simulink model "may20EOD"  (R2019b)
settings: Solver=ode4  StartTime=0.0  StopTime=inf  FixedStep=BKIN_STEP_TIME  RelTol=1e-3  EnableMultiTasking=on
StartFcn:
  |  warndlg('Dexterit-E models cannot run under simulation. Please compile your model and run it from within Dexterit-E.');set_param(bdroot,'SimulationCommand','stop')
model workspace (MAT data in the model file):
  BARRIER_ROW = 5
  BKIN_KINEMATIC_FRAME_SIZE = 400
  BKIN_STEP_TIME = 0.00025
  CIRCLE_STROKE = 10
  CIRCLE_STROKE_W = 11
  CURSOR_ROW = 2
  E_BARRIER_HIT = 6
  E_COLLISION_HIT = 7
  E_ENTER_PRESHOT_AREA = 2
  E_ENTER_START_AREA = 12
  E_EXIT = 13
  E_EXIT_PRESHOT_AREA = 10
  E_GOAL_HIT = 8
  E_GOAL_REACHED = 5
  E_NO_EVENT = 0
  E_PRESHOT_ROW = 4
  E_TARGET_OUT_OF_BOUNDS = 9
  E_TRIAL_BEGIN = 1
  E_TRIAL_ENDED = 3
  FIRST_FILL = 8
  FORCE_MULTIPLIER = 1
  F_BUMP = 1
  GOAL_ROW = 8
  GOAL_TIME = 12
  HEIGHT = 6
  INVISIBLE_FILL = 15
  LOAD_ROW = 4
  MASS_CIRCLE = 2
  MASS_RECT = 3
  PERT_DUR = 5
  PERT_RAMP = 4
  PRESHOT_ROW = 7
  PUCK_ROW = 3
  RADIUS_LOG = 4
  RADIUS_VIS = 5
  RECT_STROKE = 13
  RECT_STROKE_W = 14
  ROTATION = 7
  SECONDS = 1
  SECOND_FILL = 9
  SHOT_READY_TIME = 10
  SHOT_SET_TIME = 11
  START_HOLD_TIME = 9
  START_ROW = 6
  THIRD_FILL = 12
  TRIAL_FAILURE = 11
  WIDTH = 3
  col_x = 1
  col_y = 2
undefined symbols (not defined in the file): slselsubs
libraries: Video x7, General x3, KINARM_loads x2, KINARM_EP_loads x1, KINARM_general x1, simulink x1, slrtlib x1
(part 1 of 3)
settings Model: ModifiedComment=chris -- Wed Feb 16 09:18:30 2005 -- Version 1.1384  ModifiedHistory=Feb 16/05 - Add error repeat, add offset ramp  ExtModeArmWhenConnect=off  ExtModeLogAll=off  OrderedModelArguments=off  Creator=Chris Grebeldinger  LastModifiedBy=User
settings SolverCC: AutoInsertRateTranBlk=on
settings DataIOCC: SaveFormat=Array  SignalLoggingSaveFormat=ModelDataLogs  SaveOutput=off  SaveTime=off  ReturnWorkspaceOutputs=off  SignalLoggingName=sigsOut
settings OptimizationCC: BlockReduction=off  BooleanDataType=off  OptimizeBlockIOStorage=off  BufferReuse=off  GlobalBufferReuse=off  ExpressionFolding=off  ExpressionDepthLimit=2147483647  LocalBlockOutputs=off  InitFltsAndDblsToZero=on  LifeSpan=inf  OptimizeDataStoreBuffers=off  BusAssignmentInplaceUpdate=off
settings DebuggingCC: SaveWithParameterizedLinksMsg=none  UnderspecifiedInitializationDetection=Classic  MergeDetectMultiDrivingBlocksExec=none  SignalResolutionControl=TryResolveAllWithWarning  MultiTaskDSMMsg=warning  FcnCallInpInsideContextMsg=warning  BusObjectLabelMismatch=none  StateNameClashWarn=warning  StrictBusMsg=ErrorOnBusTreatedAsVector  SFUnexpectedBacktrackingDiag=warning  SFNoUnconditionalDefaultTransitionDiag=warning  SFExecutionAtInitializationDiag=none  ArithmeticOperatorsInVariantConditions=warning
settings HardwareCC: ProdBitPerPointer=32  ProdBitPerSizeT=32  ProdBitPerPtrDiffT=32  ProdLargestAtomicFloat=None  ProdWordSize=32  ProdLongLongMode=on  ProdHWDeviceType=Generic->32-bit x86 compatible  TargetHWDeviceType=32-bit Generic
settings ModelReferenceCC: PropagateSignalLabelsOutOfModel=off
settings SFSimCC: SimUseLocalCustomCode=off  SimParseCustomCode=off  CustomCodeUndefinedFunction=UseInterfaceOnly
settings RTWCC: Description=Simulink Real-Time  SystemTargetFile=slrt.tlc  TemplateMakefile=slrt_default_tmf  RTWUseLocalCustomCode=off  CodeExecutionProfiling=on  RTWCompilerOptimization=on
settings CodeAppCC: MaxIdLength=63  StateflowObjectComments=on
settings SimulinkRealTimeCC: TargetFcnLib=ansi_tfl_tmw.mat  GeneratePreprocessorConditionals=Disable all  PreserveStateflowLocalDataDimensions=off
settings ConfigComp: CovMetricSettings=dw  CovHtmlReporting=on  CovSaveCumulativeToWorkspaceVar=on  CovSaveSingleToWorkspaceVar=on  CovExternalEMLEnable=off

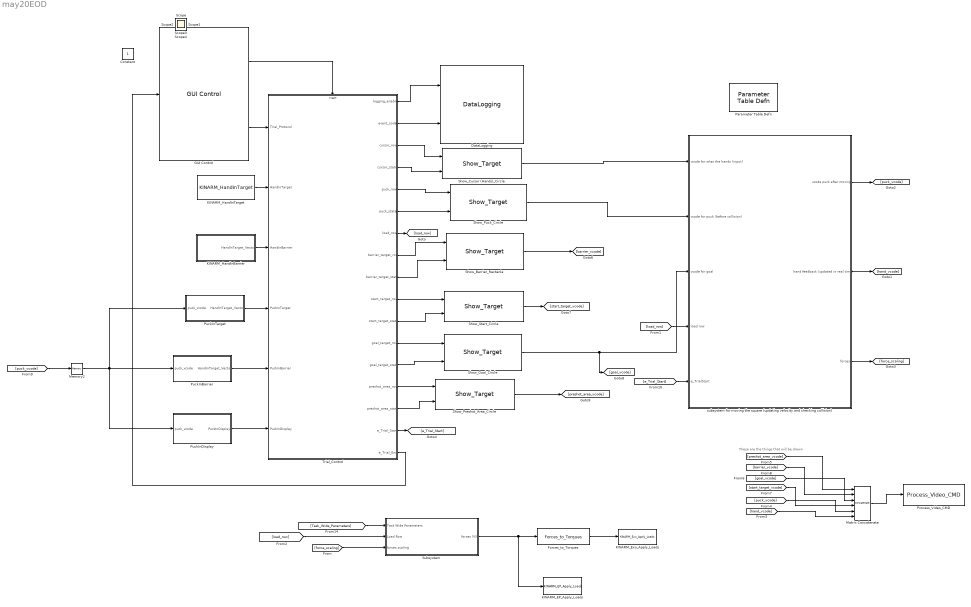
== system may20EOD ==
  note: These are the things that will be drawn
  DataLogging : General/DataLogging  log_event_codes=on  log_analog_inputs=off  show_time_remaining=off  ecat_include=on
  Forces_to_Torques : KINARM_loads/Forces_to_Torques
  GUI Control : General/GUI Control  task_version=1.0  show_repeat_trial_flag=off  use_custom_tp=off  target_type_str=Circle  Target_Type=1  XYcols=[1 2]  Vcols=3  Lcols=4  indices_padding=[0 0 0 0;0 0 0 0]  target_table_rows=64  load_table_rows=20  tp_table_rows=100
  KINARM_EP_Apply_Loads : KINARM_EP_loads/KINARM_EP_Apply_Loads  up_duration=1500  down_duration=1500  max_force=20
  KINARM_Exo_Apply_Loads : KINARM_loads/KINARM_Exo_Apply_Loads  up_duration=1500  down_duration=1500  max_torque=5  limit_motors=off
  KINARM_HandInBarrier : Subsystem  AncestorBlock=KINARM_general/KINARM_HandInTarget  mask(KINARM_HandInTarget){use_dominant_hand=on, target_type=Rectangle, num_states=1, attribcol1=[WIDTH HEIGHT ROTATION], attribcol2=[0 0 0], attribcol3=[0 0 0], attribcol4=[0 0 0], attribcol5=[0 0 0]}
      mask prompts: use_dominant_hand "Use "arm to be assessed"?"; target_type "Type of Target"; num_states "Number of Target States"; attribcol1 "State 1 Target Table Column(s)"; attribcol2 "State 2 Target Table Column(s)"; attribcol3 "State 3 Target Table Column(s)"; attribcol4 "State 4 Target Table Column(s)"; attribcol5 "State 5 Target Table Column(s)"
      mask help: This block returns a vector or array corresponding to the Target_Table rows indicating whether the specified hand is in (=1) or out (=0) of each of the targets.
      mask init:
      | block_path = gcb;  % store block path, as gcb may change with block operations
      | 
      | %%% Get the model's workspace, because it is required to evaluate constants from the Parameter Table Def'n block
      | modelName=bdroot(block_path);
      | modelWorkspace = get_param(modelName, 'ModelWorkspace');
      | 
      | %%% Handle background colours if link status changes.  
      | checkBackgroundColour(block_path, 'KINARM_general');
      | 
      | %%% create the names of the input and output ports to display on the mask
      | % Select only the desired states for output. The output port is also renamed to reflect 
      | % whether the output is a vector (in the case of a single state) or an array (of vectors, 
      | % one for each of multiple states).
      | 
      | numStates = str2double( get_param(block_path, 'num_states') );
      | 
      | if numStates == 1
      | 	set_param([block_path '/Selected States'], 'Value', '[1]');
      | 	outputname = 'HandInTarget_Vector';
      | elseif numStates == 2
      | 	set_param([block_path '/Selected States'], 'Value', '[1,2]');
      | 	outputname = 'HandInTarget_Array';
      | elseif numStates == 3
      | 	set_param([block_path '/Selected States'], 'Value', '[1,2,3]');
      | 	outputname = 'HandInTarget_Array';
      | elseif numStates == 4
      | 	set_param([block_path '/Selected States'], 'Value', '[1,2,3,4]');
      | 	outputname = 'HandInTarget_Array';
      | else
      | 	set_param([block_path '/Selected States'], 'Value', '[1,2,3,4,5]');
      | 	outputname = 'HandInTarget_Array';
      | end
      | output_block=char(find_system(gcb,'LookUnderMasks','all','FollowLinks','on','SearchDepth',1,'BlockType','Outport'));
      | set_param(output_block, 'Name', outputname);
      | 
      | 
      | %%%%%%%%%%%%%%%%%%%%%%%%%%%%%%%%%%%%%%%%%%%%%%%%%%%%%%%%%%%%%
      | %%% Check and format the input strings for the vectors of column entires
      | targetTypeStr=get_param(block_path, 'target_type');
      | 
      | switch targetTypeStr(1:3)
      | 	case 'Cir',		numCol = 1;
      | 	case 'Ell',		numCol = 3;
      |     case 'Rec',		numCol = 3;
      |     case 'Lin',		numCol = 3;
      |     case 'Tri',		numCol = 4;
      | 	otherwise,		numCol = 1;
      | end
      | 
      | for ii = 1:numStates
      | 	variableName = ['attribcol' num2str(ii)];
      | 	attribcoltext = get_param(block_path, variableName);
      | 	attribcoltext = checkUserInputVectorLength(attribcoltext, numCol);
      | 	set_param(block_path, variableName, attribcoltext);
      | end
      | 
      | for ii = 1+numStates:5
      | 	variableName = ['attribcol' num2str(ii)];
      |     if numCol == 1
      |         outstr = '[0]';
      |     else
      |         outstr = mat2str(zeros(1, numCol));
      |     end
      |     set_param(block_path, variableName, outstr);
      | end
      | 
      | %%%%%%%%%%%%%%%%%%%%%%%%%%%%%%%%%%%%%%%%%%%%%%%%%%%%%%%%%%%%%
      | %%% Create the text to show on the mask
      | numStates = str2num(get_param(block_path, 'num_states'));
      | columntext='(columns: ';
      | 
      | for ii = 1:numStates
      | 	variableName = ['attribcol' num2str(ii)];
      | 	attribcolString = get_param(block_path, variableName);
      | 	if isempty(modelWorkspace)
      | 		% if the block is part of a library, then modelWorkspace will be empty and the other code to evaluate attribcolStringEval will fail
      | 		attribcolStringEval = '3';
      | 	else
      | 		[attribcolValue, errorMessage] = BKINevalin(modelWorkspace, attribcolString);
      | 		attribcolStringEval = mat2str( attribcolValue );
      | 	end
      | 	if ii > 1
      | 		columntext = [columntext, '; ', attribcolStringEval];
      | 	else
      | 		columntext = [columntext, attribcolStringEval];
      | 	end
      | end
      | 
      | % Add formatting spaces so that the mask looks nice
      | columntext=strvcat([columntext ')'],' ', ' ');
      mask Help:
      | Used to determine if the hand (fingertip) is in any of the targets in the Target_Table.
      | <P>
      | <B><I>Use of this block requires that the DataLogging block (General library) be set to log KINARM data.</I></B>
      | 
      | <H2>Library </H2>
      | KINARM general
      | 
      | <H2>Description </H2>
      | This block returns a vector or array corresponding to the Target_Table rows indicating whether the specified hand (i.e. fingertip) is in or out of each of the targets.  Each element in the output vector or output array will be either a 0 (hand not in target) or a 1 (hand in target).
      | <P>
      | A vector is returned if only one target state is specified in each target row (see Parameters and Dialog Box), with each index of the vector corresponding to a row in the target table.  An array is returned if more than one target state is specified in a target row, with each row of the array corresponding to a target row and each column corresponding to the nth target state specified in each target row.
      | <P>
      | The output vector or array is typically used by a stateflow chart to affect behavior of the system.  Because this block returns hand-in-target information for all targets in the target table, multiple targets can be monitored at once (i.e. the Stateflow chart could have certain transitions that occur if the hand is in one target and other transitions if it is in a different target).  Likewise, because this block returns hand-in-target information for multiple states of a single target, those multiple states can be monitored simultaneously.
      | <P>
      | Because the KINARM_HandInTarget block returns information for only one hand, two copies of this block are required if information for both hands is desired.
      | <P>
      | 
      | <H2>Parameters and Dialog Box</H2>
      | <B>Use "arm to be assessed"?:</B> this checkbox determines which hand is used by this block. In Dexterit-E the operator selects the "arm to be assessed" using radio buttons.
      | When this box is checked the output of this block is derived from the hand information corresponding to the arm selection made by the operator in Dexterit-E.
      | When this box is unchecked the output of this block is derived from the contralateral arm.
      | (Note: to obtain information about both hands, then 2 separate copies of this block are required - one for each hand.)
      | <P>
      | <B>Type of Target:</B> Enter the type of target specified in the target table:
      | <P>
      | <B>Number of Target States:</B> Enter the number of target states specified in each target row.  Up to four target states are allowed per target row.
      | <P>
      | <B>State <n> Target Table Columns:</B> Enter the columns in the Target Table that specify the relevant target attributes.  Do this for each target state.
      | For a circle, enter the columns corresponding to logical radius (e.g. 4)
      | <BR>For an ellipse, enter the columns corresponding to major radius, minor radius, rotation angle (e.g. [4, 5, 6]).
      | <BR>For a rectangle, enter the columns corresponding to length, height, and rotation angle (e.g. [4, 5, 6]).
      | <BR>For a line, enter the columns corresponding to stroke width, endpoint in x, and endpoint in y (e.g. [3, 4, 5]).
      | <BR>For a triangle, enter the columns corresponding to length, height, peak offset, and rotation angle (e.g. [4, 5, 6, 7]).
      | 
      | <H2>Examples</H2>
      | <B>Example 1.</B>  Suppose a target row will be used to define 1 state for a circle type target and the radius of the visual target is the same radius to be used for determination of hand-in-target.  The related Target Table column is: column 6 = radius.  For this example, "State 1 Target Table Columns" would equal [6].
      | <P>
      | 
      | <B>Example 2.</B>  Suppose a target row will be used to define 1 state for a circle type target, but the radius of the visual target will be different than the radius to be used for determination of hand-in-target.  This option allows independent control over the size of the visual target versus the accuracy needed to be considered "in the target".  The related Target Table columns are: column 6 = radius1 (i.e. radius to target to be drawn); column 7 = radius2 (i.e. radius to be used for hand-in-target) .  For this example, "State 1 Target Table Columns" would equal [7].
      | <P>
      | <B>Example 3.</B>  Suppose a target row will be used to define 2 states for a circle type target, where the radius of the visual target will be a constant, but depending on the state of the system, one of 2 other and different radii will be used for determination of hand-in-target.  The related Target Table columns are: column 6 = radius1 (i.e. radius to target to be drawn); column 7 = radius2 (i.e. radius to be used for hand-in-target for state 1); column 8 = radius3 (i.e. radius to be used for hand-in-target for state 2).  For this example, "State 1 Target Table Columns" would equal [7], while "State 2 Target Table Columns" would equal [8].
      | <P>
      | 
      | <H2>Related Blocks </H2>
      | DataLogging
      mask TypeOptions target_type: Circle | Ellipse | Rectangle | Line | Triangle
      mask Callback target_type:
      | %%%%
      | % Because of bugs iN R2007, R2010a and R2013a (which have been reported to Mathworks), the following code
      | % is required here because in the Initialization Section it will ONLY correctly update those Mask Parameters that are hidden
      | % when the OK button is clicked (NOTE: the initialization code will correctly update all Mask Parameters when the Apply button
      | % is clicked, the bug is that it should also update everything when the OK button is clicked in the absence of an Apply click)
      | %
      | % Adding a set_param call which updates one of the mask parameters will call the initialization code to run, which "avoids"
      | % this bug. This code should be removed once Mathworks has fixed this bug.
      | 
      | temp = get_param(gcb, 'target_type');
      | set_param(gcb, 'target_type', temp);
      mask TypeOptions num_states: 1 | 2 | 3 | 4 | 5
      mask Callback num_states:
      | num_states = str2num(get_param(gcb, 'num_states'));
      | vis = get_param(gcb, 'MaskVisibilities');
      | 
      | % Select only the desired states for output. The output port is also renamed to reflect
      | % whether the output is a vector (in the case of a single state) or an array (of vectors,
      | % one for each of multiple states).
      | output_block=char(find_system(gcb, 'LookUnderMasks', 'all', 'FollowLinks', 'on', 'SearchDepth', 1, 'BlockType', 'Outport'));
      | 
      | if num_states == 1
      | % % % 	set_param([gcb '/Selected States'], 'Value', '[1]');
      | % % % 	set_param(output_block, 'Name', 'HandInTarget_Vector');
      | 	vis{5} = 'off';
      | 	vis{6} = 'off';
      | 	vis{7} = 'off';
      | 	vis{8} = 'off';
      | elseif num_states == 2
      | % % % 	set_param([gcb '/Selected States'], 'Value', '[1,2]');
      | % % % 	set_param(output_block, 'Name', 'HandInTarget_Array');
      | 	vis{5} = 'on';
      | 	vis{6} = 'off';
      | 	vis{7} = 'off';
      | 	vis{8} = 'off';
      | elseif num_states == 3
      | % % % 	set_param([gcb '/Selected States'], 'Value', '[1,2,3]');
      | % % % 	set_param(output_block, 'Name','HandInTarget_Array');
      | 	vis{5} = 'on';
      | 	vis{6} = 'on';
      | 	vis{7} = 'off';
      | 	vis{8} = 'off';
      | elseif num_states == 4
      | % % % 	set_param([gcb '/Selected States'], 'Value', '[1,2,3,4]');
      | % % % 	set_param(output_block, 'Name','HandInTarget_Array');
      | 	vis{5} = 'on';
      | 	vis{6} = 'on';
      | 	vis{7} = 'on';
      | 	vis{8} = 'off';
      | else
      | % % % 	set_param([gcb '/Selected States'], 'Value', '[1,2,3,4,5]');
      | % % % 	set_param(output_block, 'Name', 'HandInTarget_Array');
      | 	vis{5} = 'on';
      | 	vis{6} = 'on';
      | 	vis{7} = 'on';
      | 	vis{8} = 'on';
      | end
      | set_param(gcb, 'MaskVisibilities', vis);
      mask Display:
      | disp(columntext);
      | port_label('output',1,outputname);
  KINARM_HandInTarget : KINARM_general/KINARM_HandInTarget  use_dominant_hand=on  target_type=Circle  num_states=1  attribcol1=[RADIUS_LOG]  attribcol2=[0]  attribcol3=[0]  attribcol4=[0]  attribcol5=[0]
  Matrix Concatenate : Concatenate  NumInputs=6  Mode=Multidimensional array
  Memory2 : Memory
  Parameter Table Defn : General/Parameter Table Defn  ShowInLibBrowser=0
  Process_Video_CMD : Video/Process_Video_CMD  video_delay=0
  PuckInBarrier : Subsystem  AncestorBlock=KINARM_general/KINARM_HandInTarget  mask(KINARM_HandInTarget){use_dominant_hand=on, target_type=Rectangle, num_states=1, attribcol1=[WIDTH HEIGHT ROTATION], attribcol2=[0 0 0], attribcol3=[0 0 0], attribcol4=[0 0 0], attribcol5=[0 0 0]}
      mask prompts: use_dominant_hand "Use "arm to be assessed"?"; target_type "Type of Target"; num_states "Number of Target States"; attribcol1 "State 1 Target Table Column(s)"; attribcol2 "State 2 Target Table Column(s)"; attribcol3 "State 3 Target Table Column(s)"; attribcol4 "State 4 Target Table Column(s)"; attribcol5 "State 5 Target Table Column(s)"
      mask help: This block returns a vector or array corresponding to the Target_Table rows indicating whether the specified hand is in (=1) or out (=0) of each of the targets.
      mask init: same as may20EOD/KINARM_HandInBarrier
      mask Help:
      | Used to determine if the hand (fingertip) is in any of the targets in the Target_Table.
      | <P>
      | <B><I>Use of this block requires that the DataLogging block (General library) be set to log KINARM data.</I></B>
      | 
      | <H2>Library </H2>
      | KINARM general
      | 
      | <H2>Description </H2>
      | This block returns a vector or array corresponding to the Target_Table rows indicating whether the specified hand (i.e. fingertip) is in or out of each of the targets.  Each element in the output vector or output array will be either a 0 (hand not in target) or a 1 (hand in target).
      | <P>
      | A vector is returned if only one target state is specified in each target row (see Parameters and Dialog Box), with each index of the vector corresponding to a row in the target table.  An array is returned if more than one target state is specified in a target row, with each row of the array corresponding to a target row and each column corresponding to the nth target state specified in each target row.
      | <P>
      | The output vector or array is typically used by a stateflow chart to affect behavior of the system.  Because this block returns hand-in-target information for all targets in the target table, multiple targets can be monitored at once (i.e. the Stateflow chart could have certain transitions that occur if the hand is in one target and other transitions if it is in a different target).  Likewise, because this block returns hand-in-target information for multiple states of a single target, those multiple states can be monitored simultaneously.
      | <P>
      | Because the KINARM_HandInTarget block returns information for only one hand, two copies of this block are required if information for both hands is desired.
      | <P>
      | 
      | <H2>Parameters and Dialog Box</H2>
      | <B>Use "arm to be assessed"?:</B> this checkbox determines which hand is used by this block. In Dexterit-E the operator selects the "arm to be assessed" using radio buttons.
      | When this box is checked the output of this block is derived from the hand information corresponding to the arm selection made by the operator in Dexterit-E.
      | When this box is unchecked the output of this block is derived from the contralateral arm.
      | (Note: to obtain information about both hands, then 2 separate copies of this block are required - one for each hand.)
      | <P>
      | <B>Type of Target:</B> Enter the type of target specified in the target table:
      | <P>
      | <B>Number of Target States:</B> Enter the number of target states specified in each target row.  Up to four target states are allowed per target row.
      | <P>
      | <B>State <n> Target Table Columns:</B> Enter the columns in the Target Table that specify the relevant target attributes.  Do this for each target state.
      | For a circle, enter the columns corresponding to logical radius (e.g. 4)
      | <BR>For an ellipse, enter the columns corresponding to major radius, minor radius, rotation angle (e.g. [4, 5, 6]).
      | <BR>For a rectangle, enter the columns corresponding to length, height, and rotation angle (e.g. [4, 5, 6]).
      | <BR>For a line, enter the columns corresponding to stroke width, endpoint in x, and endpoint in y (e.g. [3, 4, 5]).
      | <BR>For a triangle, enter the columns corresponding to length, height, peak offset, and rotation angle (e.g. [4, 5, 6, 7]).
      | 
      | <H2>Examples</H2>
      | <B>Example 1.</B>  Suppose a target row will be used to define 1 state for a circle type target and the radius of the visual target is the same radius to be used for determination of hand-in-target.  The related Target Table column is: column 6 = radius.  For this example, "State 1 Target Table Columns" would equal [6].
      | <P>
      | 
      | <B>Example 2.</B>  Suppose a target row will be used to define 1 state for a circle type target, but the radius of the visual target will be different than the radius to be used for determination of hand-in-target.  This option allows independent control over the size of the visual target versus the accuracy needed to be considered "in the target".  The related Target Table columns are: column 6 = radius1 (i.e. radius to target to be drawn); column 7 = radius2 (i.e. radius to be used for hand-in-target) .  For this example, "State 1 Target Table Columns" would equal [7].
      | <P>
      | <B>Example 3.</B>  Suppose a target row will be used to define 2 states for a circle type target, where the radius of the visual target will be a constant, but depending on the state of the system, one of 2 other and different radii will be used for determination of hand-in-target.  The related Target Table columns are: column 6 = radius1 (i.e. radius to target to be drawn); column 7 = radius2 (i.e. radius to be used for hand-in-target for state 1); column 8 = radius3 (i.e. radius to be used for hand-in-target for state 2).  For this example, "State 1 Target Table Columns" would equal [7], while "State 2 Target Table Columns" would equal [8].
      | <P>
      | 
      | <H2>Related Blocks </H2>
      | DataLogging
      mask TypeOptions target_type: Circle | Ellipse | Rectangle | Line | Triangle
      mask Callback target_type:
      | %%%%
      | % Because of bugs iN R2007, R2010a and R2013a (which have been reported to Mathworks), the following code
      | % is required here because in the Initialization Section it will ONLY correctly update those Mask Parameters that are hidden
      | % when the OK button is clicked (NOTE: the initialization code will correctly update all Mask Parameters when the Apply button
      | % is clicked, the bug is that it should also update everything when the OK button is clicked in the absence of an Apply click)
      | %
      | % Adding a set_param call which updates one of the mask parameters will call the initialization code to run, which "avoids"
      | % this bug. This code should be removed once Mathworks has fixed this bug.
      | 
      | temp = get_param(gcb, 'target_type');
      | set_param(gcb, 'target_type', temp);
      mask TypeOptions num_states: 1 | 2 | 3 | 4 | 5
      mask Callback num_states:
      | num_states = str2num(get_param(gcb, 'num_states'));
      | vis = get_param(gcb, 'MaskVisibilities');
      | 
      | % Select only the desired states for output. The output port is also renamed to reflect
      | % whether the output is a vector (in the case of a single state) or an array (of vectors,
      | % one for each of multiple states).
      | output_block=char(find_system(gcb, 'LookUnderMasks', 'all', 'FollowLinks', 'on', 'SearchDepth', 1, 'BlockType', 'Outport'));
      | 
      | if num_states == 1
      | % % % 	set_param([gcb '/Selected States'], 'Value', '[1]');
      | % % % 	set_param(output_block, 'Name', 'HandInTarget_Vector');
      | 	vis{5} = 'off';
      | 	vis{6} = 'off';
      | 	vis{7} = 'off';
      | 	vis{8} = 'off';
      | elseif num_states == 2
      | % % % 	set_param([gcb '/Selected States'], 'Value', '[1,2]');
      | % % % 	set_param(output_block, 'Name', 'HandInTarget_Array');
      | 	vis{5} = 'on';
      | 	vis{6} = 'off';
      | 	vis{7} = 'off';
      | 	vis{8} = 'off';
      | elseif num_states == 3
      | % % % 	set_param([gcb '/Selected States'], 'Value', '[1,2,3]');
      | % % % 	set_param(output_block, 'Name','HandInTarget_Array');
      | 	vis{5} = 'on';
      | 	vis{6} = 'on';
      | 	vis{7} = 'off';
      | 	vis{8} = 'off';
      | elseif num_states == 4
      | % % % 	set_param([gcb '/Selected States'], 'Value', '[1,2,3,4]');
      | % % % 	set_param(output_block, 'Name','HandInTarget_Array');
      | 	vis{5} = 'on';
      | 	vis{6} = 'on';
      | 	vis{7} = 'on';
      | 	vis{8} = 'off';
      | else
      | % % % 	set_param([gcb '/Selected States'], 'Value', '[1,2,3,4,5]');
      | % % % 	set_param(output_block, 'Name', 'HandInTarget_Array');
      | 	vis{5} = 'on';
      | 	vis{6} = 'on';
      | 	vis{7} = 'on';
      | 	vis{8} = 'on';
      | end
      | set_param(gcb, 'MaskVisibilities', vis);
      mask Display:
      | disp(columntext);
      | port_label('output',1,outputname);
  PuckInDisplay : Subsystem
  PuckInTarget : Subsystem  AncestorBlock=KINARM_general/KINARM_HandInTarget  mask(KINARM_HandInTarget){use_dominant_hand=on, target_type=Circle, num_states=1, attribcol1=[RADIUS_LOG], attribcol2=[0], attribcol3=[0], attribcol4=[0], attribcol5=[0]}
      mask prompts: use_dominant_hand "Use "arm to be assessed"?"; target_type "Type of Target"; num_states "Number of Target States"; attribcol1 "State 1 Target Table Column(s)"; attribcol2 "State 2 Target Table Column(s)"; attribcol3 "State 3 Target Table Column(s)"; attribcol4 "State 4 Target Table Column(s)"; attribcol5 "State 5 Target Table Column(s)"
      mask help: This block returns a vector or array corresponding to the Target_Table rows indicating whether the specified hand is in (=1) or out (=0) of each of the targets.
      mask init: same as may20EOD/KINARM_HandInBarrier
      mask Help:
      | Used to determine if the hand (fingertip) is in any of the targets in the Target_Table.
      | <P>
      | <B><I>Use of this block requires that the DataLogging block (General library) be set to log KINARM data.</I></B>
      | 
      | <H2>Library </H2>
      | KINARM general
      | 
      | <H2>Description </H2>
      | This block returns a vector or array corresponding to the Target_Table rows indicating whether the specified hand (i.e. fingertip) is in or out of each of the targets.  Each element in the output vector or output array will be either a 0 (hand not in target) or a 1 (hand in target).
      | <P>
      | A vector is returned if only one target state is specified in each target row (see Parameters and Dialog Box), with each index of the vector corresponding to a row in the target table.  An array is returned if more than one target state is specified in a target row, with each row of the array corresponding to a target row and each column corresponding to the nth target state specified in each target row.
      | <P>
      | The output vector or array is typically used by a stateflow chart to affect behavior of the system.  Because this block returns hand-in-target information for all targets in the target table, multiple targets can be monitored at once (i.e. the Stateflow chart could have certain transitions that occur if the hand is in one target and other transitions if it is in a different target).  Likewise, because this block returns hand-in-target information for multiple states of a single target, those multiple states can be monitored simultaneously.
      | <P>
      | Because the KINARM_HandInTarget block returns information for only one hand, two copies of this block are required if information for both hands is desired.
      | <P>
      | 
      | <H2>Parameters and Dialog Box</H2>
      | <B>Use "arm to be assessed"?:</B> this checkbox determines which hand is used by this block. In Dexterit-E the operator selects the "arm to be assessed" using radio buttons.
      | When this box is checked the output of this block is derived from the hand information corresponding to the arm selection made by the operator in Dexterit-E.
      | When this box is unchecked the output of this block is derived from the contralateral arm.
      | (Note: to obtain information about both hands, then 2 separate copies of this block are required - one for each hand.)
      | <P>
      | <B>Type of Target:</B> Enter the type of target specified in the target table:
      | <P>
      | <B>Number of Target States:</B> Enter the number of target states specified in each target row.  Up to four target states are allowed per target row.
      | <P>
      | <B>State <n> Target Table Columns:</B> Enter the columns in the Target Table that specify the relevant target attributes.  Do this for each target state.
      | For a circle, enter the columns corresponding to logical radius (e.g. 4)
      | <BR>For an ellipse, enter the columns corresponding to major radius, minor radius, rotation angle (e.g. [4, 5, 6]).
      | <BR>For a rectangle, enter the columns corresponding to length, height, and rotation angle (e.g. [4, 5, 6]).
      | <BR>For a line, enter the columns corresponding to stroke width, endpoint in x, and endpoint in y (e.g. [3, 4, 5]).
      | <BR>For a triangle, enter the columns corresponding to length, height, peak offset, and rotation angle (e.g. [4, 5, 6, 7]).
      | 
      | <H2>Examples</H2>
      | <B>Example 1.</B>  Suppose a target row will be used to define 1 state for a circle type target and the radius of the visual target is the same radius to be used for determination of hand-in-target.  The related Target Table column is: column 6 = radius.  For this example, "State 1 Target Table Columns" would equal [6].
      | <P>
      | 
      | <B>Example 2.</B>  Suppose a target row will be used to define 1 state for a circle type target, but the radius of the visual target will be different than the radius to be used for determination of hand-in-target.  This option allows independent control over the size of the visual target versus the accuracy needed to be considered "in the target".  The related Target Table columns are: column 6 = radius1 (i.e. radius to target to be drawn); column 7 = radius2 (i.e. radius to be used for hand-in-target) .  For this example, "State 1 Target Table Columns" would equal [7].
      | <P>
      | <B>Example 3.</B>  Suppose a target row will be used to define 2 states for a circle type target, where the radius of the visual target will be a constant, but depending on the state of the system, one of 2 other and different radii will be used for determination of hand-in-target.  The related Target Table columns are: column 6 = radius1 (i.e. radius to target to be drawn); column 7 = radius2 (i.e. radius to be used for hand-in-target for state 1); column 8 = radius3 (i.e. radius to be used for hand-in-target for state 2).  For this example, "State 1 Target Table Columns" would equal [7], while "State 2 Target Table Columns" would equal [8].
      | <P>
      | 
      | <H2>Related Blocks </H2>
      | DataLogging
      mask TypeOptions target_type: Circle | Ellipse | Rectangle | Line | Triangle
      mask Callback target_type:
      | %%%%
      | % Because of bugs iN R2007, R2010a and R2013a (which have been reported to Mathworks), the following code
      | % is required here because in the Initialization Section it will ONLY correctly update those Mask Parameters that are hidden
      | % when the OK button is clicked (NOTE: the initialization code will correctly update all Mask Parameters when the Apply button
      | % is clicked, the bug is that it should also update everything when the OK button is clicked in the absence of an Apply click)
      | %
      | % Adding a set_param call which updates one of the mask parameters will call the initialization code to run, which "avoids"
      | % this bug. This code should be removed once Mathworks has fixed this bug.
      | 
      | temp = get_param(gcb, 'target_type');
      | set_param(gcb, 'target_type', temp);
      mask TypeOptions num_states: 1 | 2 | 3 | 4 | 5
      mask Callback num_states:
      | num_states = str2num(get_param(gcb, 'num_states'));
      | vis = get_param(gcb, 'MaskVisibilities');
      | 
      | % Select only the desired states for output. The output port is also renamed to reflect
      | % whether the output is a vector (in the case of a single state) or an array (of vectors,
      | % one for each of multiple states).
      | output_block=char(find_system(gcb, 'LookUnderMasks', 'all', 'FollowLinks', 'on', 'SearchDepth', 1, 'BlockType', 'Outport'));
      | 
      | if num_states == 1
      | % % % 	set_param([gcb '/Selected States'], 'Value', '[1]');
      | % % % 	set_param(output_block, 'Name', 'HandInTarget_Vector');
      | 	vis{5} = 'off';
      | 	vis{6} = 'off';
      | 	vis{7} = 'off';
      | 	vis{8} = 'off';
      | elseif num_states == 2
      | % % % 	set_param([gcb '/Selected States'], 'Value', '[1,2]');
      | % % % 	set_param(output_block, 'Name', 'HandInTarget_Array');
      | 	vis{5} = 'on';
      | 	vis{6} = 'off';
      | 	vis{7} = 'off';
      | 	vis{8} = 'off';
      | elseif num_states == 3
      | % % % 	set_param([gcb '/Selected States'], 'Value', '[1,2,3]');
      | % % % 	set_param(output_block, 'Name','HandInTarget_Array');
      | 	vis{5} = 'on';
      | 	vis{6} = 'on';
      | 	vis{7} = 'off';
      | 	vis{8} = 'off';
      | elseif num_states == 4
      | % % % 	set_param([gcb '/Selected States'], 'Value', '[1,2,3,4]');
      | % % % 	set_param(output_block, 'Name','HandInTarget_Array');
      | 	vis{5} = 'on';
      | 	vis{6} = 'on';
      | 	vis{7} = 'on';
      | 	vis{8} = 'off';
      | else
      | % % % 	set_param([gcb '/Selected States'], 'Value', '[1,2,3,4,5]');
      | % % % 	set_param(output_block, 'Name', 'HandInTarget_Array');
      | 	vis{5} = 'on';
      | 	vis{6} = 'on';
      | 	vis{7} = 'on';
      | 	vis{8} = 'on';
      | end
      | set_param(gcb, 'MaskVisibilities', vis);
      mask Display:
      | disp(columntext);
      | port_label('output',1,outputname);
  Show_Barrier_Rectanle : Video/Show_Target  target_type=Rectangle  num_states=2  attribcol1=[FIRST_FILL RECT_STROKE RECT_STROKE_W WIDTH HEIGHT ROTATION]  attribcol2=[SECOND_FILL RECT_STROKE RECT_STROKE_W WIDTH HEIGHT ROTATION]  attribcol3=[0 0 0 0 0 0]  attribcol4=[0 0 0 0 0 0]  attribcol5=[0 0 0 0 0 0]  stateindices_padding=[0 0 0 0 0;0 0 0 0 0;0 0 0 0 0;0 0 0 0 0;0 0 0 0 0]  source=dialog  opacity=100  target_display=Both subject and operator displays  num_col=6
  Show_Cursor (Hands)_Circle : Video/Show_Target  target_type=Circle  num_states=2  attribcol1=[FIRST_FILL CIRCLE_STROKE CIRCLE_STROKE_W WIDTH]  attribcol2=[SECOND_FILL CIRCLE_STROKE CIRCLE_STROKE_W WIDTH]  attribcol3=[0 0 0 0]  attribcol4=[0 0 0 0]  attribcol5=[0 0 0 0]  stateindices_padding=[0 0 0 0 0 0 0;0 0 0 0 0 0 0;0 0 0 0 0 0 0;0 0 0 0 0 0 0;0 0 0 0 0 0 0]  source=dialog  opacity=100  target_display=Both subject and operator displays  num_col=4
  Show_Goal_Circle : Video/Show_Target  target_type=Circle  num_states=3  attribcol1=[INVISIBLE_FILL RECT_STROKE RECT_STROKE_W WIDTH]  attribcol2=[FIRST_FILL RECT_STROKE RECT_STROKE_W WIDTH]  attribcol3=[SECOND_FILL RECT_STROKE RECT_STROKE_W WIDTH]  attribcol4=[0 0 0 0]  attribcol5=[0 0 0 0]  stateindices_padding=[0 0 0 0 0 0 0;0 0 0 0 0 0 0;0 0 0 0 0 0 0;0 0 0 0 0 0 0;0 0 0 0 0 0 0]  source=dialog  opacity=100  target_display=Both subject and operator displays  num_col=4
  Show_Preshot_Area_Circle : Video/Show_Target  target_type=Circle  num_states=3  attribcol1=[INVISIBLE_FILL CIRCLE_STROKE CIRCLE_STROKE_W WIDTH]  attribcol2=[FIRST_FILL CIRCLE_STROKE CIRCLE_STROKE_W WIDTH]  attribcol3=[SECOND_FILL CIRCLE_STROKE CIRCLE_STROKE_W WIDTH]  attribcol4=[0 0 0 0]  attribcol5=[0 0 0 0]  stateindices_padding=[0 0 0 0 0 0 0;0 0 0 0 0 0 0;0 0 0 0 0 0 0;0 0 0 0 0 0 0;0 0 0 0 0 0 0]  source=dialog  opacity=100  target_display=Both subject and operator displays  num_col=4
  Show_Puck_Circle : Video/Show_Target  target_type=Circle  num_states=3  attribcol1=[INVISIBLE_FILL RECT_STROKE RECT_STROKE_W WIDTH]  attribcol2=[FIRST_FILL RECT_STROKE RECT_STROKE_W WIDTH]  attribcol3=[SECOND_FILL RECT_STROKE RECT_STROKE_W WIDTH]  attribcol4=[0 0 0 0]  attribcol5=[0 0 0 0]  stateindices_padding=[0 0 0 0 0 0 0;0 0 0 0 0 0 0;0 0 0 0 0 0 0;0 0 0 0 0 0 0;0 0 0 0 0 0 0]  source=dialog  opacity=100  target_display=Both subject and operator displays  num_col=4
  Show_Start_Circle : Video/Show_Target  target_type=Circle  num_states=3  attribcol1=[INVISIBLE_FILL CIRCLE_STROKE CIRCLE_STROKE_W WIDTH]  attribcol2=[FIRST_FILL CIRCLE_STROKE CIRCLE_STROKE_W WIDTH]  attribcol3=[SECOND_FILL CIRCLE_STROKE CIRCLE_STROKE_W WIDTH]  attribcol4=[0 0 0 0]  attribcol5=[0 0 0 0]  stateindices_padding=[0 0 0 0 0 0 0;0 0 0 0 0 0 0;0 0 0 0 0 0 0;0 0 0 0 0 0 0;0 0 0 0 0 0 0]  source=dialog  opacity=100  target_display=Both subject and operator displays  num_col=4
  Subsystem : Subsystem
  Trial_Control : Stateflow chart  TreatAsAtomicUnit=on
  subsystem for moving the square (updating velocity and checking collision) : Subsystem
  Constant : Constant  IOType=siggen
  Scope{,1..4} (5 alike) : Scope
  wires:
  Trial_Control/3(cursor_row) -> Show_Cursor (Hands)_Circle/1
  Trial_Control/5(puck_row) -> Show_Puck_Circle/1
  Trial_Control/6(puck_state) -> Show_Puck_Circle/2
  Forces_to_Torques/1 -> KINARM_Exo_Apply_Loads/1
  Trial_Control/1(logging_enable) -> DataLogging/1
  Trial_Control/7(load_row) -> [load_row]
  Trial_Control/17(e_Trial_End) -> GUI Control/1
  Trial_Control/4(cursor_state) -> Show_Cursor (Hands)_Circle/2
  GUI Control/1 -> Trial_Control/Trigger
  Matrix Concatenate/1 -> Process_Video_CMD/1
  Show_Cursor (Hands)_Circle/1 -> subsystem for moving the square (updating velocity and checking collision)/1(vcode for what the hands (input))
  Show_Puck_Circle/1 -> subsystem for moving the square (updating velocity and checking collision)/2(vcode for puck (before collision))
  subsystem for moving the square (updating velocity and checking collision)/1(vcode puck after moving) -> [puck_vcode]
  subsystem for moving the square (updating velocity and checking collision)/3(forces) -> [force_scaling]
  subsystem for moving the square (updating velocity and checking collision)/2(hand feedback (updated in real time)) -> [hand_vcode]
  Trial_Control/2(event_code) -> DataLogging/2
  Subsystem/1(forces (N)) -> KINARM_EP_Apply_Loads/1, Forces_to_Torques/1
  [Task_Wide_Parameters] -> Subsystem/1(Task Wide Parameters)
  [load_row] -> Subsystem/2(Load Row)
  [force_scaling] -> Subsystem/3(forces scaling)
  [load_row] -> subsystem for moving the square (updating velocity and checking collision)/4(load row)
  Trial_Control/8(barrier_target_row) -> Show_Barrier_Rectanle/1
  Trial_Control/9(barrier_target_state) -> Show_Barrier_Rectanle/2
  Trial_Control/10(start_target_row) -> Show_Start_Circle/1
  Trial_Control/11(start_target_state) -> Show_Start_Circle/2
  Trial_Control/12(goal_target_row) -> Show_Goal_Circle/1
  Trial_Control/13(goal_target_state) -> Show_Goal_Circle/2
  KINARM_HandInTarget/1 -> Trial_Control/2(HandInTarget)
  GUI Control/2 -> Trial_Control/1(Trial_Protocol)
  Show_Barrier_Rectanle/1 -> [barrier_vcode]
  Show_Preshot_Area_Circle/1 -> [preshot_area_vcode]
  Show_Goal_Circle/1 -> [goal_vcode], subsystem for moving the square (updating velocity and checking collision)/3(vcode for goal)
  Show_Start_Circle/1 -> [start_target_vcode]
  Trial_Control/15(preshot_area_state) -> Show_Preshot_Area_Circle/2
  Trial_Control/14(preshot_area_row) -> Show_Preshot_Area_Circle/1
  [hand_vcode] -> Matrix Concatenate/6
  [puck_vcode] -> Matrix Concatenate/5
  [preshot_area_vcode] -> Matrix Concatenate/1
  [barrier_vcode] -> Matrix Concatenate/2
  [goal_vcode] -> Matrix Concatenate/3
  [start_target_vcode] -> Matrix Concatenate/4
  KINARM_HandInBarrier/1(HandInTarget_Vector) -> Trial_Control/3(HandInBarrier)
  [puck_vcode] -> Memory2/1
  PuckInTarget/1(HandInTarget_Vector) -> Trial_Control/4(PuckInTarget)
  Memory2/1 -> PuckInDisplay/1(puck_vcode), PuckInTarget/1(puck_vcode), PuckInBarrier/1(puck_vcode)
  Trial_Control/16(e_Trial_Start) -> [e_Trial_Start]
  [e_Trial_Start] -> subsystem for moving the square (updating velocity and checking collision)/5(e_TrialStart)
  PuckInBarrier/1(HandInTarget_Vector) -> Trial_Control/5(PuckInBarrier)
  PuckInDisplay/1(PuckInDisplay) -> Trial_Control/6(PuckInDisplay)

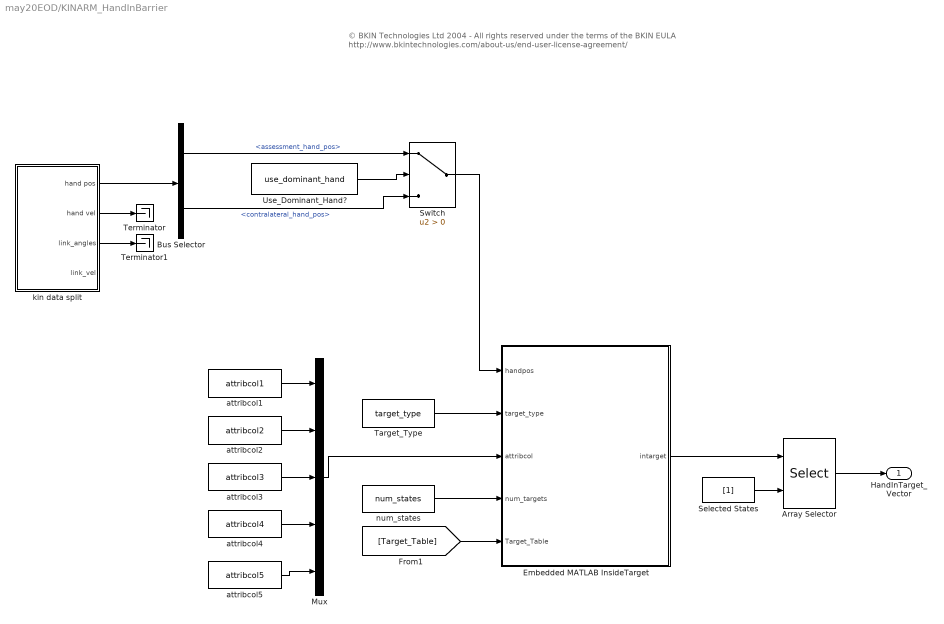
== system may20EOD/KINARM_HandInBarrier ==
  note: © BKIN Technologies Ltd 2004  - All rights reserved under the terms of the BKIN EULA
      | http://www.bkintechnologies.com/about-us/end-user-license-agreement/
  Array Selector : Selector  NumberOfDimensions=2  InputPortWidth=3  IndexOptions=Select all,Index vector (port)  Indices=-1,1  OutputSizes=slselsubs([(-2),(-2)],1),slselsubs([(-2),(-2)],2)
  Bus Selector : BusSelector  OutputSignals=assessment_hand_pos,contralateral_hand_pos
  Embedded MATLAB InsideTarget : MATLAB Function  TreatAsAtomicUnit=on
      settings: RTWSystemCode=Nonreusable function  RTWFileNameOpts=Use function name
  Mux : Mux  Inputs=5
  Selected States : Constant  Value=[1]
  Switch : Switch  Criteria=u2 > Threshold
  Target_Type : Constant  Value=target_type
  Terminator : Terminator
  Terminator1 : Terminator
  Use_Dominant_Hand? : Constant  Value=use_dominant_hand
  attribcol1 : Constant  Value=attribcol1
  attribcol2 : Constant  Value=attribcol2
  attribcol3 : Constant  Value=attribcol3
  attribcol4 : Constant  Value=attribcol4
  attribcol5 : Constant  Value=attribcol5
  kin data split : Subsystem
  num_states : Constant  Value=num_states
  HandInTarget_Vector : Outport
  wires:
  Selected States/1 -> Array Selector/2
  num_states/1 -> Embedded MATLAB InsideTarget/4(num_targets)
  Mux/1 -> Embedded MATLAB InsideTarget/3(attribcol)
  attribcol4/1 -> Mux/4
  attribcol3/1 -> Mux/3
  attribcol2/1 -> Mux/2
  attribcol1/1 -> Mux/1
  Target_Type/1 -> Embedded MATLAB InsideTarget/2(target_type)
  Array Selector/1 -> HandInTarget_Vector/1
  [Target_Table] -> Embedded MATLAB InsideTarget/5(Target_Table)
  Embedded MATLAB InsideTarget/1(intarget) -> Array Selector/1
  attribcol5/1 -> Mux/5
  kin data split/1(hand pos) -> Bus Selector/1
  Use_Dominant_Hand?/1 -> Switch/2
  Bus Selector/1 -> Switch/1  "<assessment_hand_pos>"
  Bus Selector/2 -> Switch/3  "<contralateral_hand_pos>"
  kin data split/2(hand vel) -> Terminator/1
  kin data split/3(link_angles) -> Terminator1/1
  Switch/1 -> Embedded MATLAB InsideTarget/1(handpos)

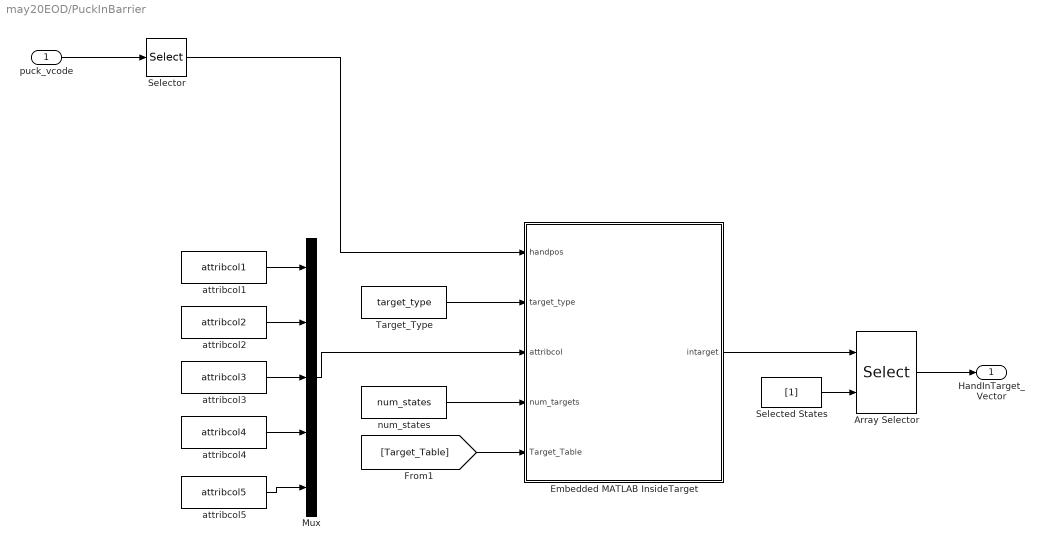
== system may20EOD/PuckInBarrier ==
  puck_vcode : Inport  PortDimensions=[1,70]
  Array Selector : Selector  NumberOfDimensions=2  InputPortWidth=3  IndexOptions=Select all,Index vector (port)  Indices=-1,1  OutputSizes=slselsubs([(-2),(-2)],1),slselsubs([(-2),(-2)],2)
  Embedded MATLAB InsideTarget : MATLAB Function  TreatAsAtomicUnit=on
      settings: RTWSystemCode=Nonreusable function  RTWFileNameOpts=Use function name
  Mux : Mux  Inputs=5
  Selected States : Constant  Value=[1]
  Selector : Selector  NumberOfDimensions=2  InputPortWidth=3  IndexOptions=Index vector (dialog),Index vector (dialog)  Indices=1,[3,4]  OutputSizes=1,1
  Target_Type : Constant  Value=target_type
  attribcol1 : Constant  Value=attribcol1
  attribcol2 : Constant  Value=attribcol2
  attribcol3 : Constant  Value=attribcol3
  attribcol4 : Constant  Value=attribcol4
  attribcol5 : Constant  Value=attribcol5
  num_states : Constant  Value=num_states
  HandInTarget_Vector : Outport
  wires:
  Selected States/1 -> Array Selector/2
  num_states/1 -> Embedded MATLAB InsideTarget/4(num_targets)
  Mux/1 -> Embedded MATLAB InsideTarget/3(attribcol)
  attribcol4/1 -> Mux/4
  attribcol3/1 -> Mux/3
  attribcol2/1 -> Mux/2
  attribcol1/1 -> Mux/1
  Target_Type/1 -> Embedded MATLAB InsideTarget/2(target_type)
  Array Selector/1 -> HandInTarget_Vector/1
  [Target_Table] -> Embedded MATLAB InsideTarget/5(Target_Table)
  Embedded MATLAB InsideTarget/1(intarget) -> Array Selector/1
  attribcol5/1 -> Mux/5
  Selector/1 -> Embedded MATLAB InsideTarget/1(handpos)
  puck_vcode/1 -> Selector/1

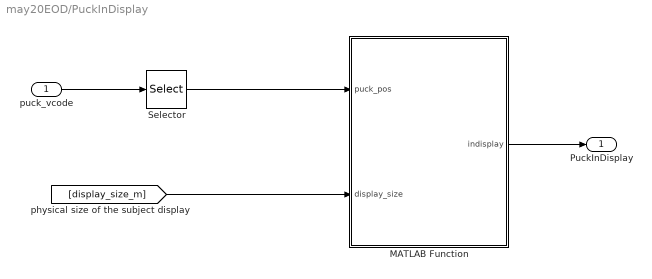
== system may20EOD/PuckInDisplay ==
  puck_vcode : Inport  PortDimensions=[1,70]
  MATLAB Function : MATLAB Function  TreatAsAtomicUnit=on
  Selector : Selector  NumberOfDimensions=2  InputPortWidth=3  IndexOptions=Index vector (dialog),Index vector (dialog)  Indices=1,[3,4]  OutputSizes=1,1
  PuckInDisplay : Outport
  wires:
  Selector/1 -> MATLAB Function/1(puck_pos)
  MATLAB Function/1(indisplay) -> PuckInDisplay/1
  puck_vcode/1 -> Selector/1
  [display_size_m] -> MATLAB Function/2(display_size)

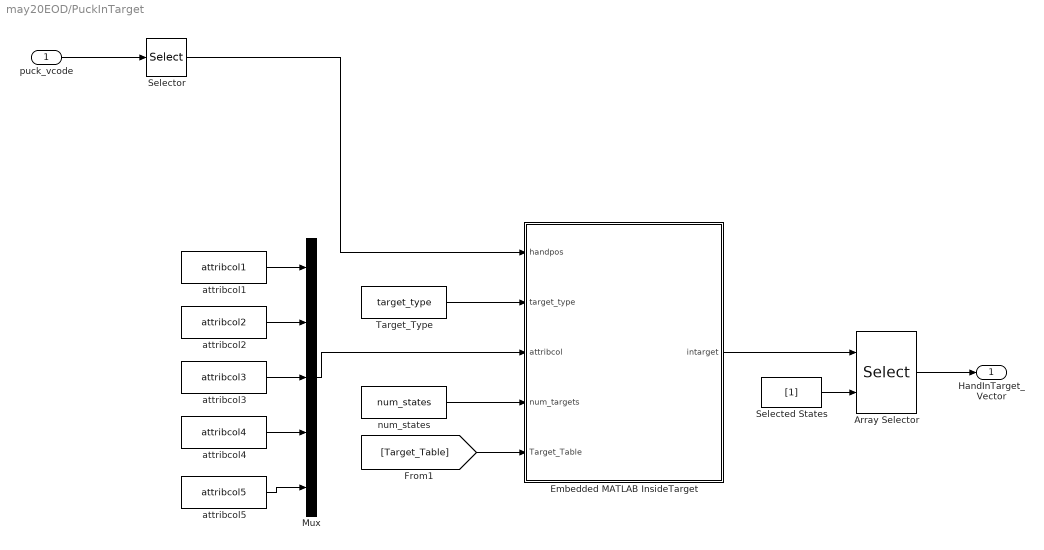
== system may20EOD/PuckInTarget ==
  puck_vcode : Inport  PortDimensions=[1,70]
  Array Selector : Selector  NumberOfDimensions=2  InputPortWidth=3  IndexOptions=Select all,Index vector (port)  Indices=-1,1  OutputSizes=slselsubs([(-2),(-2)],1),slselsubs([(-2),(-2)],2)
  Embedded MATLAB InsideTarget : MATLAB Function  TreatAsAtomicUnit=on
      settings: RTWSystemCode=Nonreusable function  RTWFileNameOpts=Use function name
  Mux : Mux  Inputs=5
  Selected States : Constant  Value=[1]
  Selector : Selector  NumberOfDimensions=2  InputPortWidth=3  IndexOptions=Index vector (dialog),Index vector (dialog)  Indices=1,[3,4]  OutputSizes=1,1
  Target_Type : Constant  Value=target_type
  attribcol1 : Constant  Value=attribcol1
  attribcol2 : Constant  Value=attribcol2
  attribcol3 : Constant  Value=attribcol3
  attribcol4 : Constant  Value=attribcol4
  attribcol5 : Constant  Value=attribcol5
  num_states : Constant  Value=num_states
  HandInTarget_Vector : Outport
  wires:
  Selected States/1 -> Array Selector/2
  num_states/1 -> Embedded MATLAB InsideTarget/4(num_targets)
  Mux/1 -> Embedded MATLAB InsideTarget/3(attribcol)
  attribcol4/1 -> Mux/4
  attribcol3/1 -> Mux/3
  attribcol2/1 -> Mux/2
  attribcol1/1 -> Mux/1
  Target_Type/1 -> Embedded MATLAB InsideTarget/2(target_type)
  Array Selector/1 -> HandInTarget_Vector/1
  [Target_Table] -> Embedded MATLAB InsideTarget/5(Target_Table)
  Embedded MATLAB InsideTarget/1(intarget) -> Array Selector/1
  attribcol5/1 -> Mux/5
  Selector/1 -> Embedded MATLAB InsideTarget/1(handpos)
  puck_vcode/1 -> Selector/1
